simulink model "CEngDsT"  (R2020b)
settings: configuration reference "cs_ert" (kept outside this file)
settings Model: DataDictionary=CEngDsT.sldd  EnableAccessToBaseWorkspace=off  Creator=zhoutinglin  LastModifiedBy=zhoutinglin
settings ConfigSetRef: SourceName=cs_ert

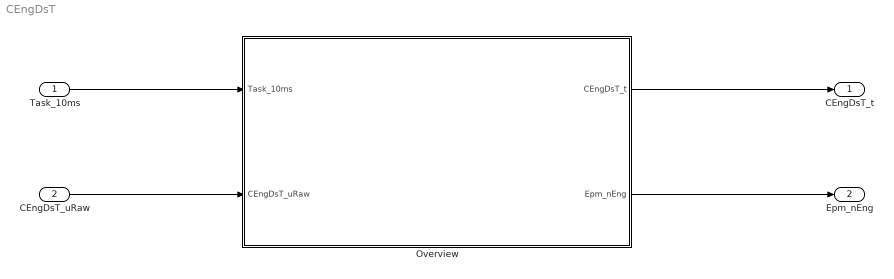
== system CEngDsT ==
  Task_10ms : Inport  OutputFunctionCall=on
  CEngDsT_uRaw : Inport  Port=2
  Overview : Subsystem
  CEngDsT_t : Outport
  Epm_nEng : Outport  Port=2
  wires:
  Task_10ms/1 -> Overview/1(Task_10ms)
  CEngDsT_uRaw/1 -> Overview/2(CEngDsT_uRaw)
  Overview/1(CEngDsT_t) -> CEngDsT_t/1
  Overview/2(Epm_nEng) -> Epm_nEng/1

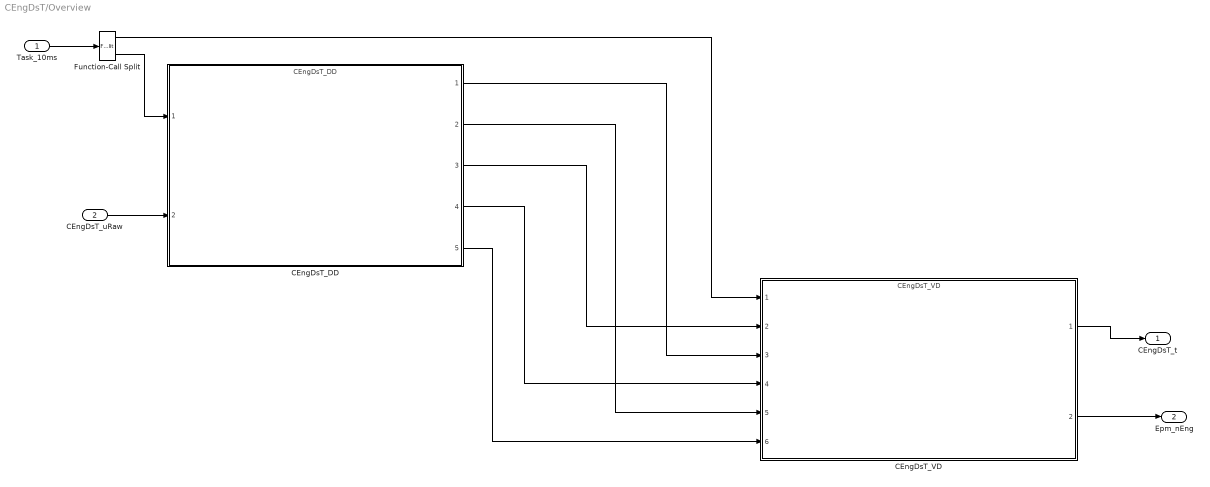
== system CEngDsT/Overview ==
  Task_10ms : Inport
  CEngDsT_uRaw : Inport  Port=2
  CEngDsT_DD : ModelReference  ModelNameDialog=CEngDsT_DD  SimulationMode=Normal  ScheduleRates=on  ModelReferenceVersion=1.57
  CEngDsT_VD : ModelReference  ModelNameDialog=CEngDsT_VD  SimulationMode=Normal  ScheduleRates=on  ModelReferenceVersion=6.4
  Function-Call Split : FunctionCallSplit  IconShape=distinctive  NumOutputPorts=2  OutputPortLayout=default
  CEngDsT_t : Outport  VectorParamsAs1DForOutWhenUnconnected=off
  Epm_nEng : Outport  Port=2
  wires:
  CEngDsT_VD/1 -> CEngDsT_t/1
  Task_10ms/1 -> Function-Call Split/1
  CEngDsT_uRaw/1 -> CEngDsT_DD/2
  Function-Call Split/2 -> CEngDsT_DD/1
  Function-Call Split/1 -> CEngDsT_VD/1
  CEngDsT_DD/3 -> CEngDsT_VD/2
  CEngDsT_DD/1 -> CEngDsT_VD/3
  CEngDsT_DD/4 -> CEngDsT_VD/4
  CEngDsT_DD/2 -> CEngDsT_VD/5
  CEngDsT_DD/5 -> CEngDsT_VD/6
  CEngDsT_VD/2 -> Epm_nEng/1
